simulink model "ME655_Grp7_Simulink_Latest"  (R2022b)
settings: Solver=FixedStepAuto  StartTime=0.0  StopTime=60  FixedStep=.003  RelTol=1e-3
values from neighbouring files (symbols this model uses):
  A = [1 T;0 1]    [ME655_Grp7_MATLAB.m]
  Bh = 62.8318530718    [ME655_Lect09_VL3_Data.mat]
  dt_active_control = 10    [ME655_Grp7_MATLAB.m]
  g = 9.81    [ME655_Lect09_VL3_Data.mat]
  h = 2.5*N    (= 200)    [ME655_Grp7_MATLAB.m]
  H = eye(2)    [ME655_Grp7_MATLAB.m]
  IHC = 1.16793611779    [ME655_Lect09_VL3_Data.mat]
  IRC = 0.090069676016    [ME655_Lect09_VL3_Data.mat]
  k = -K*RhipAvg + LhipAvg    [ME655_Grp7_MATLAB.m]
  K = Sp*C*inv(Sh)    [ME655_Grp7_MATLAB.m]
  Kh = 986.960440109    [ME655_Lect09_VL3_Data.mat]
  lambda = .95    (= 0.95)    [ME655_Grp7_MATLAB.m]
  LH = 0.426438    [ME655_Lect09_VL3_Data.mat]
  Lhip_pos0 = Lhip_pos(1)    [ME655_Grp7_MATLAB.m]
  Lhip_vel0 = Lhip_vel(1)    [ME655_Grp7_MATLAB.m]
  LR = 0.2474    [ME655_Lect09_VL3_Data.mat]
  M = 6    [ME655_Grp7_MATLAB.m]
  mH = 12.075    [ME655_Lect09_VL3_Data.mat]
  mR = 7.7284    [ME655_Lect09_VL3_Data.mat]
  N = 80    [ME655_Grp7_MATLAB.m]
  nu = .5    (= 0.5)    [ME655_Grp7_MATLAB.m]
  Q = G*G'*var(Lhip_acc(train_indices(:)))    [ME655_Grp7_MATLAB.m]
  R = [var(Lhip_pred(:,1)-Lhip_pos_train) 0;0 var(Lhip_pred(:,2)-Lhip_vel_train)]    [ME655_Grp7_MATLAB.m]
  t_start = 5.0    (= 5)    [ME655_Grp7_MATLAB.m]
  Tau_h_max = 30    [ME655_Grp7_MATLAB.m]
undefined symbols (not defined in the file or in its folder): theta_0, theta_d0
settings Model: Creator=Damiano  LastModifiedBy=peeratienthong
settings SolverCC: AlgebraicLoopSolver=TrustRegion
settings DataIOCC: ReturnWorkspaceOutputs=off
settings DebuggingCC: UnconnectedInputMsg=warning  UnconnectedOutputMsg=warning  UnconnectedLineMsg=warning  SFMachineParentedDataDiag=warning  ArithmeticOperatorsInVariantConditions=warning
settings ModelReferenceCC: EnableRefExpFcnMdlSchedulingChecks=on
settings SFSimCC: SimUseLocalCustomCode=off  CustomCodeUndefinedFunction=UseInterfaceOnly
settings RTWCC: RTWUseLocalCustomCode=off  DLArmComputeVersion=19.05
settings CodeAppCC: StateflowObjectComments=on

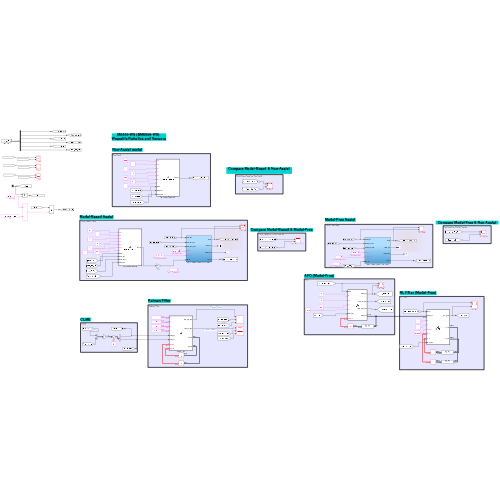
[thumbnail: Simulink's stored preview of the top-level diagram]
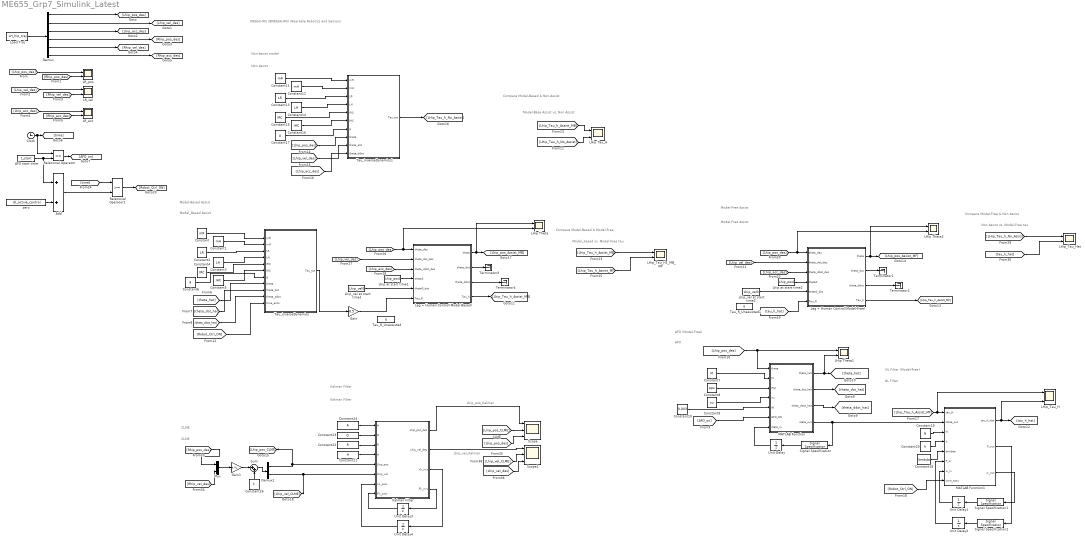
== system ME655_Grp7_Simulink_Latest ==
  note: Model_based vs. Model-Free tau
  note: Model-Free Assist
  note: NL Filter
  note: AFO
  note: Model_Based Assist
  note: Kalman Filter
  note: CLME
  note: Non Assist
  note: Model-Base Assist vs. Non Assist
  note: Lhip_pos_Kalman
  note: Lhip_vel_Kalman
  note: ME655-WS (BME656-WS)
      | Wearable Robotics and Sensors
  note: Non-Assist model
  note: Model-Based Assist
  note: Compare Model-Based & Non-Assist
  note: Model-Free Assist
  note: AFO (Model-Free)
  note: NL Filter (Model-Free)
  note: Compare Model-Based & Model-Free
  note: CLME
  note: Kalman Filter
  note: Compare Model-Free & Non Assist
  note: Non Assist vs. Model-Free tau
  AFO start time : Constant  Value=t_start
  Add : Sum
  Clock : Clock
  Constant : Constant  Value=mR
  Constant1 : Constant  Value=mH
  Constant10 : Constant  Value=0.003
  Constant11 : Constant  Value=mR
  Constant12 : Constant  Value=mH
  Constant13 : Constant  Value=LR
  Constant14 : Constant  Value=LH
  Constant15 : Constant  Value=IRC
  Constant16 : Constant  Value=IHC
  Constant17 : Constant  Value=g
  Constant18 : Constant  Value=lambda
  Constant19 : Constant  Value=N
  Constant2 : Constant  Value=LR
  Constant20 : Constant  Value=h
  Constant21 : Constant  Value=H
  Constant22 : Constant  Value=R
  Constant23 : Constant  Value=Q
  Constant24 : Constant  Value=A
  Constant26 : Constant  Value=k
  Constant3 : Constant  Value=LH
  Constant4 : Constant  Value=IRC
  Constant5 : Constant  Value=IHC
  Constant6 : Constant  Value=g
  Constant7 : Constant  Value=M
  Constant8 : Constant  Value=eps
  Constant9 : Constant  Value=nu
  Demux : Demux  Outputs=6
  Demux1 : Demux  Outputs=2
  Gain : Gain  Gain=0.5
  Gain1 : Gain  Gain=K  Multiplication=Matrix(K*u)
  Kalman Filter : MATLAB Function  TreatAsAtomicUnit=on
  LHip Tau_H : Scope  NumInputPorts=2
  LHip Theta : Scope  NumInputPorts=2
  LHip Theta1 : Scope  NumInputPorts=2
  LHip Theta2 : Scope  NumInputPorts=2
  LHip_Tau_H : Scope  NumInputPorts=2
  LHip_Tau_H1_MB_MF : Scope  NumInputPorts=2
  LHip_Tau_Hat : Scope  NumInputPorts=2
  "LR_acc " : Scope  NumInputPorts=2
  LR_pos : Scope  NumInputPorts=2
  LR_vel : Scope  NumInputPorts=2
  Leg + Human Control(Model-Based) : Subsystem
  Leg + Human Control(Model-Free) : Subsystem
  Lhip at start time1 : Constant  Value=Lhip_pos0
  Lhip at start time2 : Constant  Value=Lhip_pos0
  Lhip_vel at start time1 : Constant  Value=Lhip_vel0
  Lhip_vel at start time2 : Constant  Value=Lhip_vel0
  Load Traj : FromWorkspace  VariableName=LH_hip_traj
  MATLAB Function : MATLAB Function  TreatAsAtomicUnit=on
  MATLAB Function1 : MATLAB Function  TreatAsAtomicUnit=on
  Mux : Mux  Inputs=2
  Relational Operator : RelationalOperator  OutDataTypeStr=boolean  RndMeth=Simplest  InputSameDT=off
  Relational Operator1 : RelationalOperator  OutDataTypeStr=boolean  RndMeth=Simplest  InputSameDT=off
  Scope : Scope  NumInputPorts=3
  Scope1 : Scope  NumInputPorts=3
  Signal Specification : SignalSpecification  Dimensions=[1,14]
  Signal Specification1 : SignalSpecification  Dimensions=[1,N]
  Signal Specification2 : SignalSpecification  Dimensions=[1,N]
  Sum : Sum  Inputs=|++
  Tau_R_Unassisted : Constant  Value=0
  Tau_R_Unassisted1 : Constant  Value=0
  Tau_inverseDynamics : MATLAB Function  TreatAsAtomicUnit=on
  Tau_inverseDynamics1 : MATLAB Function  TreatAsAtomicUnit=on
  Terminator{1..4} (4 alike) : Terminator
  Unit Delay : UnitDelay  InitialCondition=[[pi/2,pi/2,pi/2,pi/2,pi/2,pi/2],[0,0,0,0,0,0], 3*pi/2, 0]  SampleTime=-1  HasFrameUpgradeWarning=on
  Unit Delay1 : UnitDelay  InitialCondition=zeros(1,N)  SampleTime=-1  HasFrameUpgradeWarning=on
  Unit Delay2 : UnitDelay  InitialCondition=ones(1,N)  SampleTime=-1  HasFrameUpgradeWarning=on
  Unit Delay3 : UnitDelay  InitialCondition=eye(2)  SampleTime=-1  HasFrameUpgradeWarning=on
  Unit Delay4 : UnitDelay  InitialCondition=[0;0]  SampleTime=-1  HasFrameUpgradeWarning=on
  zero : Constant  Value=dt_active_control
  wires:
  Load Traj/1 -> Demux/1
  Demux/6 -> [Rhip_acc_des]
  Demux/4 -> [Rhip_pos_des]
  Demux/5 -> [Rhip_vel_des]
  [Lhip_pos_des] -> LR_pos/1
  [Rhip_pos_des] -> LR_pos/2
  [Lhip_vel_des] -> LR_vel/1
  [Rhip_vel_des] -> LR_vel/2
  [Lhip_acc_des] -> "LR_acc "/1
  [Rhip_acc_des] -> "LR_acc "/2
  Clock/1 -> Relational Operator/1, [time]
  Relational Operator/1 -> [AFO_on]
  [time] -> Relational Operator1/1
  AFO start time/1 -> Add/1, Relational Operator/2
  Add/1 -> Relational Operator1/2
  zero/1 -> Add/2
  [Lhip_acc_des] -> Leg + Human Control(Model-Based)/3(theta_ddot_des)
  Leg + Human Control(Model-Based)/3(theta_ddot) -> Terminator4/1
  Lhip_vel at start time1/1 -> Leg + Human Control(Model-Based)/5(theta0_dot)
  Leg + Human Control(Model-Based)/2(theta_dot) -> Terminator3/1
  [Lhip_vel_des] -> Leg + Human Control(Model-Based)/2(theta_dot_des)
  Lhip at start time1/1 -> Leg + Human Control(Model-Based)/4(theta0)
  Leg + Human Control(Model-Based)/4(Tau_h) -> [Lhip_Tau_h_Assist_MB]
  [Lhip_pos_des] -> Leg + Human Control(Model-Based)/1(theta_des), LHip Theta/2
  Relational Operator1/1 -> [Robot_Ctrl_ON]
  Demux/1 -> [Lhip_pos_des]
  Demux/2 -> [Lhip_vel_des]
  Demux/3 -> [Lhip_acc_des]
  [theta_hat] -> Tau_inverseDynamics/8(theta)
  [theta_dot_hat] -> Tau_inverseDynamics/9(theta_dot)
  [theta_ddot_hat] -> Tau_inverseDynamics/10(theta_ddot)
  Constant/1 -> Tau_inverseDynamics/1(mR)
  Constant1/1 -> Tau_inverseDynamics/2(mH)
  Constant2/1 -> Tau_inverseDynamics/3(LR)
  Constant3/1 -> Tau_inverseDynamics/4(LH)
  Constant4/1 -> Tau_inverseDynamics/5(IRC)
  Constant5/1 -> Tau_inverseDynamics/6(IHC)
  Constant6/1 -> Tau_inverseDynamics/7(g)
  [AFO_on] -> MATLAB Function/6(AFO_ON)
  Constant9/1 -> MATLAB Function/4(nu)
  Constant8/1 -> MATLAB Function/3(esp)
  Constant7/1 -> MATLAB Function/2(M)
  [Lhip_pos_des] -> LHip Theta1/1, MATLAB Function/1(theta)
  MATLAB Function/1(theta_hat) -> [theta_hat], LHip Theta1/2
  Leg + Human Control(Model-Based)/1(theta) -> LHip Theta/1, [Lhip_pos_Assist_MB]
  Constant10/1 -> MATLAB Function/5(dt)
  MATLAB Function/3(theta_ddot_hat) -> [theta_ddot_hat]
  MATLAB Function/2(theta_dot_hat) -> [theta_dot_hat]
  Unit Delay/1 -> MATLAB Function/7(state_in)
  Signal Specification/1 -> Unit Delay/1
  MATLAB Function/4(state_out) -> MATLAB Function1/2(state_out), Signal Specification/1
  [Robot_Ctrl_ON] -> Tau_inverseDynamics/11(time_activ)
  [Lhip_pos_des] -> Tau_inverseDynamics1/8(theta)
  Constant13/1 -> Tau_inverseDynamics1/3(LR)
  Constant11/1 -> Tau_inverseDynamics1/1(mR)
  Constant12/1 -> Tau_inverseDynamics1/2(mH)
  Constant14/1 -> Tau_inverseDynamics1/4(LH)
  Constant15/1 -> Tau_inverseDynamics1/5(IRC)
  [Lhip_acc_des] -> Tau_inverseDynamics1/10(theta_ddot)
  Constant17/1 -> Tau_inverseDynamics1/7(g)
  [Lhip_vel_des] -> Tau_inverseDynamics1/9(theta_dot)
  Constant16/1 -> Tau_inverseDynamics1/6(IHC)
  Tau_inverseDynamics1/1(Tau_tot) -> [LHip_Tau_h_No_Assist]
  Tau_inverseDynamics/1(Tau_tot) -> Gain/1
  [Lhip_Tau_h_Assist_MB] -> LHip Tau_H/1
  [LHip_Tau_h_No_Assist] -> LHip Tau_H/2
  Signal Specification1/1 -> Unit Delay1/1
  Signal Specification2/1 -> Unit Delay2/1
  MATLAB Function1/3(w_out) -> Signal Specification1/1
  MATLAB Function1/2(P_out) -> Signal Specification2/1
  Unit Delay1/1 -> MATLAB Function1/7(w_in)
  Unit Delay2/1 -> MATLAB Function1/6(P_in)
  Constant19/1 -> MATLAB Function1/3(N)
  Constant20/1 -> MATLAB Function1/4(h)
  Constant18/1 -> MATLAB Function1/5(lambda)
  [Lhip_Tau_h_Assist_MF] -> LHip_Tau_H/1, MATLAB Function1/1(tau_H)
  MATLAB Function1/1(tau_h_hat) -> LHip_Tau_H/2, [tau_h_hat]
  [Robot_Ctrl_ON] -> MATLAB Function1/8(time_activ)
  Leg + Human Control(Model-Free)/4(Tau_h) -> [Lhip_Tau_h_Assist_MF]
  Leg + Human Control(Model-Free)/2(theta_dot) -> Terminator1/1
  Leg + Human Control(Model-Free)/3(theta_ddot) -> Terminator2/1
  [Lhip_vel_des] -> Leg + Human Control(Model-Free)/2(theta_dot_des)
  Lhip at start time2/1 -> Leg + Human Control(Model-Free)/4(theta0)
  Leg + Human Control(Model-Free)/1(theta) -> LHip Theta2/1, [Lhip_pos_Assist_MF]
  [Lhip_acc_des] -> Leg + Human Control(Model-Free)/3(theta_ddot_des)
  Lhip_vel at start time2/1 -> Leg + Human Control(Model-Free)/5(theta0_dot)
  [Lhip_pos_des] -> Leg + Human Control(Model-Free)/1(theta_des), LHip Theta2/2
  [Lhip_Tau_h_Assist_MF] -> LHip_Tau_H1_MB_MF/2
  [Lhip_Tau_h_Assist_MB] -> LHip_Tau_H1_MB_MF/1
  Constant24/1 -> Kalman Filter/1(A)
  Constant23/1 -> Kalman Filter/2(Q)
  Constant22/1 -> Kalman Filter/3(R)
  Constant21/1 -> Kalman Filter/4(H)
  [Rhip_pos_des] -> Mux/1
  [Rhip_vel_des] -> Mux/2
  Mux/1 -> Gain1/1
  Gain1/1 -> Sum/1
  Constant26/1 -> Sum/2
  Sum/1 -> Demux1/1
  Demux1/1 -> Kalman Filter/5(Lhip_pos), [Lhip_pos_CLME]
  Demux1/2 -> [Lhip_vel_CLME], Kalman Filter/6(Lhip_vel)
  Unit Delay3/1 -> Kalman Filter/8(Pk_prev)
  Kalman Filter/4(Pk_nxt) -> Unit Delay3/1
  Kalman Filter/3(xk_nxt) -> Unit Delay4/1
  Unit Delay4/1 -> Kalman Filter/7(xk_prev)
  Kalman Filter/1(Lhip_pos_des) -> Scope/1
  Kalman Filter/2(Lhip_vel_des) -> Scope1/1
  [Lhip_pos_des] -> Scope/3
  [Lhip_vel_des] -> Scope1/3
  [Lhip_pos_CLME] -> Scope/2
  [Lhip_vel_CLME] -> Scope1/2
  Gain/1 -> Leg + Human Control(Model-Based)/6(Tau_R)
  [LHip_Tau_h_No_Assist] -> LHip_Tau_Hat/1
  [tau_h_hat] -> LHip_Tau_Hat/2
  [tau_h_hat] -> Leg + Human Control(Model-Free)/6(Tau_R)

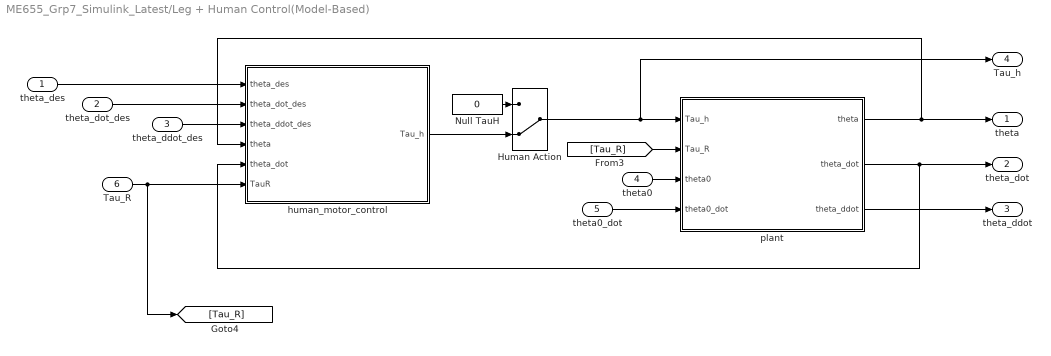
== system ME655_Grp7_Simulink_Latest/Leg + Human Control(Model-Based) ==
  theta_des : Inport
  theta_dot_des : Inport  Port=2
  theta_ddot_des : Inport  Port=3
  theta0 : Inport  Port=4
  theta0_dot : Inport  Port=5
  Tau_R : Inport  Port=6
  Human Action : ManualSwitch  CurrentSetting=0
  Null TauH : Constant  Value=0
  human_motor_control : Subsystem
  plant : Subsystem
  theta : Outport  PortDimensions=[1,1]  VectorParamsAs1DForOutWhenUnconnected=off
  theta_dot : Outport  Port=2  PortDimensions=[1,1]  VectorParamsAs1DForOutWhenUnconnected=off
  theta_ddot : Outport  Port=3  PortDimensions=[1,1]  VectorParamsAs1DForOutWhenUnconnected=off
  Tau_h : Outport  Port=4  PortDimensions=[1,1]  VectorParamsAs1DForOutWhenUnconnected=off
  wires:
  theta_des/1 -> human_motor_control/1(theta_des)
  theta_dot_des/1 -> human_motor_control/2(theta_dot_des)
  theta0/1 -> plant/3(theta0)
  theta0_dot/1 -> plant/4(theta0_dot)
  [Tau_R] -> plant/2(Tau_R)
  plant/1(theta) -> theta/1, human_motor_control/4(theta)
  plant/2(theta_dot) -> human_motor_control/5(theta_dot), theta_dot/1
  plant/3(theta_ddot) -> theta_ddot/1
  theta_ddot_des/1 -> human_motor_control/3(theta_ddot_des)
  human_motor_control/1(Tau_h) -> Human Action/2
  Human Action/1 -> Tau_h/1, plant/1(Tau_h)
  Null TauH/1 -> Human Action/1
  Tau_R/1 -> [Tau_R], human_motor_control/6(TauR)

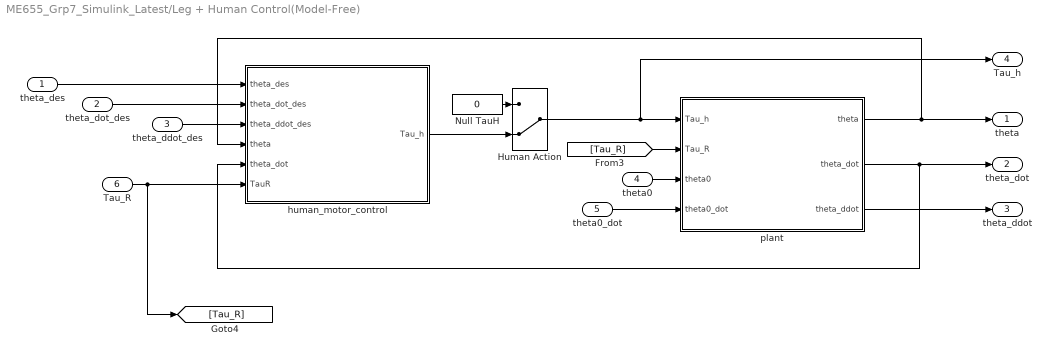
== system ME655_Grp7_Simulink_Latest/Leg + Human Control(Model-Free) ==
  theta_des : Inport
  theta_dot_des : Inport  Port=2
  theta_ddot_des : Inport  Port=3
  theta0 : Inport  Port=4
  theta0_dot : Inport  Port=5
  Tau_R : Inport  Port=6
  Human Action : ManualSwitch  CurrentSetting=0
  Null TauH : Constant  Value=0
  human_motor_control : Subsystem
  plant : Subsystem
  theta : Outport  PortDimensions=[1,1]  VectorParamsAs1DForOutWhenUnconnected=off
  theta_dot : Outport  Port=2  PortDimensions=[1,1]  VectorParamsAs1DForOutWhenUnconnected=off
  theta_ddot : Outport  Port=3  PortDimensions=[1,1]  VectorParamsAs1DForOutWhenUnconnected=off
  Tau_h : Outport  Port=4  PortDimensions=[1,1]  VectorParamsAs1DForOutWhenUnconnected=off
  wires:
  theta_des/1 -> human_motor_control/1(theta_des)
  theta_dot_des/1 -> human_motor_control/2(theta_dot_des)
  theta0/1 -> plant/3(theta0)
  theta0_dot/1 -> plant/4(theta0_dot)
  [Tau_R] -> plant/2(Tau_R)
  plant/1(theta) -> theta/1, human_motor_control/4(theta)
  plant/2(theta_dot) -> human_motor_control/5(theta_dot), theta_dot/1
  plant/3(theta_ddot) -> theta_ddot/1
  theta_ddot_des/1 -> human_motor_control/3(theta_ddot_des)
  human_motor_control/1(Tau_h) -> Human Action/2
  Human Action/1 -> Tau_h/1, plant/1(Tau_h)
  Null TauH/1 -> Human Action/1
  Tau_R/1 -> [Tau_R], human_motor_control/6(TauR)

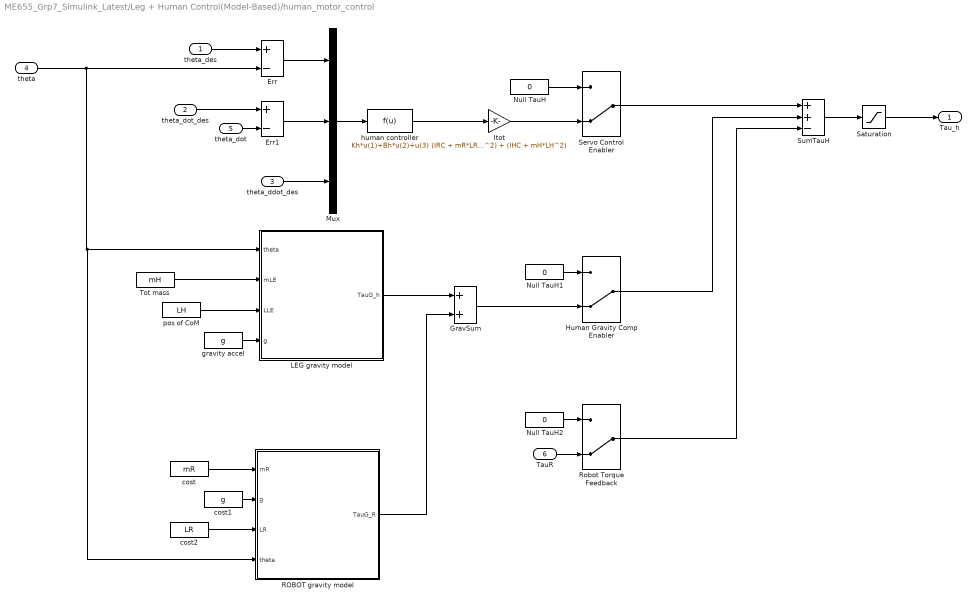
== system ME655_Grp7_Simulink_Latest/Leg + Human Control(Model-Based)/human_motor_control ==
  theta_des : Inport
  theta_dot_des : Inport  Port=2
  theta_ddot_des : Inport  Port=3
  theta : Inport  Port=4
  theta_dot : Inport  Port=5
  TauR : Inport  Port=6
  Err : Sum  Inputs=+-
  Err1 : Sum  Inputs=+-
  GravSum : Sum
  Human Gravity Comp Enabler : ManualSwitch  CurrentSetting=0
  Itot : Gain  Gain=(IRC + mR*LR^2) + (IHC + mH*LH^2)
  LEG gravity model : MATLAB Function  TreatAsAtomicUnit=on
  Mux : Mux  Inputs=3
  Null TauH : Constant  Value=0
  Null TauH1 : Constant  Value=0
  Null TauH2 : Constant  Value=0
  ROBOT gravity model : MATLAB Function  TreatAsAtomicUnit=on
  Robot Torque Feedback : ManualSwitch  CurrentSetting=0
  Saturation : Saturate  UpperLimit=Tau_h_max  LowerLimit=-Tau_h_max
  Servo Control Enabler : ManualSwitch  CurrentSetting=0
  SumTauH : Sum  Inputs=++-
  Tot mass : Constant  Value=mH
  cost : Constant  Value=mR
  cost1 : Constant  Value=g
  cost2 : Constant  Value=LR
  gravity accel : Constant  Value=g
  human controller : Fcn  Expr=Kh*u(1)+Bh*u(2)+u(3)
  pos of CoM : Constant  Value=LH
  Tau_h : Outport  PortDimensions=[1,1]  VectorParamsAs1DForOutWhenUnconnected=off
  wires:
  theta_des/1 -> Err/1
  theta_dot_des/1 -> Err1/1
  theta_dot/1 -> Err1/2
  Err/1 -> Mux/1
  Err1/1 -> Mux/2
  Mux/1 -> human controller/1
  theta_ddot_des/1 -> Mux/3
  gravity accel/1 -> LEG gravity model/4(g)
  Tot mass/1 -> LEG gravity model/2(mLE)
  pos of CoM/1 -> LEG gravity model/3(LLE)
  Null TauH/1 -> Servo Control Enabler/1
  Null TauH1/1 -> Human Gravity Comp Enabler/1
  Human Gravity Comp Enabler/1 -> SumTauH/2
  SumTauH/1 -> Saturation/1
  human controller/1 -> Itot/1
  Servo Control Enabler/1 -> SumTauH/1
  Saturation/1 -> Tau_h/1
  Itot/1 -> Servo Control Enabler/2
  Null TauH2/1 -> Robot Torque Feedback/1
  TauR/1 -> Robot Torque Feedback/2
  Robot Torque Feedback/1 -> SumTauH/3
  theta/1 -> ROBOT gravity model/4(theta), LEG gravity model/1(theta), Err/2
  ROBOT gravity model/1(TauG_R) -> GravSum/2
  cost2/1 -> ROBOT gravity model/3(LR)
  cost/1 -> ROBOT gravity model/1(mR)
  cost1/1 -> ROBOT gravity model/2(g)
  LEG gravity model/1(TauG_h) -> GravSum/1
  GravSum/1 -> Human Gravity Comp Enabler/2

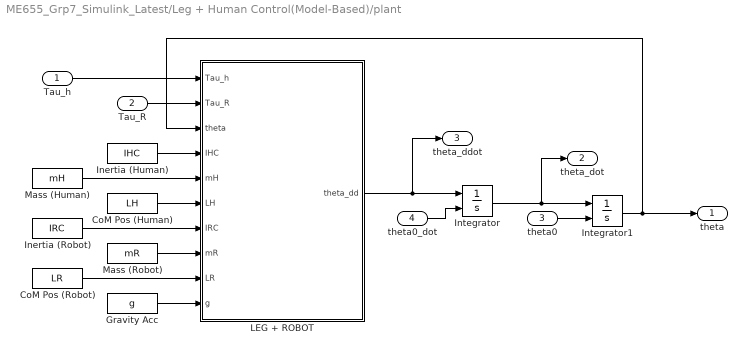
== system ME655_Grp7_Simulink_Latest/Leg + Human Control(Model-Based)/plant ==
  Tau_h : Inport
  Tau_R : Inport  Port=2
  theta0 : Inport  Port=3
  theta0_dot : Inport  Port=4
  CoM Pos (Human) : Constant  Value=LH
  CoM Pos (Robot) : Constant  Value=LR
  Gravity Acc : Constant  Value=g
  Inertia (Human) : Constant  Value=IHC
  Inertia (Robot) : Constant  Value=IRC
  Integrator : Integrator  InitialConditionSource=external  InitialCondition=theta_d0
  Integrator1 : Integrator  InitialConditionSource=external  InitialCondition=theta_0
  LEG + ROBOT : MATLAB Function  TreatAsAtomicUnit=on
  Mass (Human) : Constant  Value=mH
  Mass (Robot) : Constant  Value=mR
  theta : Outport  PortDimensions=[1,1]  VectorParamsAs1DForOutWhenUnconnected=off
  theta_dot : Outport  Port=2  PortDimensions=[1,1]  VectorParamsAs1DForOutWhenUnconnected=off
  theta_ddot : Outport  Port=3  PortDimensions=[1,1]  VectorParamsAs1DForOutWhenUnconnected=off
  wires:
  Tau_h/1 -> LEG + ROBOT/1(Tau_h)
  Tau_R/1 -> LEG + ROBOT/2(Tau_R)
  LEG + ROBOT/1(theta_dd) -> theta_ddot/1, Integrator/1
  Integrator/1 -> theta_dot/1, Integrator1/1
  theta0_dot/1 -> Integrator/2
  theta0/1 -> Integrator1/2
  Integrator1/1 -> LEG + ROBOT/3(theta), theta/1
  Inertia (Human)/1 -> LEG + ROBOT/4(IHC)
  Mass (Human)/1 -> LEG + ROBOT/5(mH)
  CoM Pos (Human)/1 -> LEG + ROBOT/6(LH)
  Gravity Acc/1 -> LEG + ROBOT/10(g)
  Mass (Robot)/1 -> LEG + ROBOT/8(mR)
  CoM Pos (Robot)/1 -> LEG + ROBOT/9(LR)
  Inertia (Robot)/1 -> LEG + ROBOT/7(IRC)

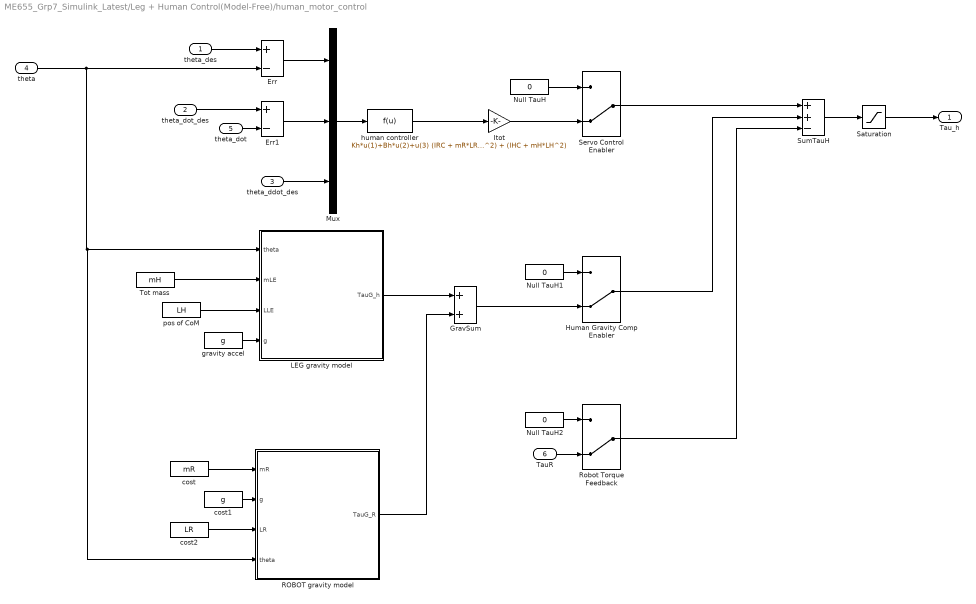
== system ME655_Grp7_Simulink_Latest/Leg + Human Control(Model-Free)/human_motor_control ==
  theta_des : Inport
  theta_dot_des : Inport  Port=2
  theta_ddot_des : Inport  Port=3
  theta : Inport  Port=4
  theta_dot : Inport  Port=5
  TauR : Inport  Port=6
  Err : Sum  Inputs=+-
  Err1 : Sum  Inputs=+-
  GravSum : Sum
  Human Gravity Comp Enabler : ManualSwitch  CurrentSetting=0
  Itot : Gain  Gain=(IRC + mR*LR^2) + (IHC + mH*LH^2)
  LEG gravity model : MATLAB Function  TreatAsAtomicUnit=on
  Mux : Mux  Inputs=3
  Null TauH : Constant  Value=0
  Null TauH1 : Constant  Value=0
  Null TauH2 : Constant  Value=0
  ROBOT gravity model : MATLAB Function  TreatAsAtomicUnit=on
  Robot Torque Feedback : ManualSwitch  CurrentSetting=0
  Saturation : Saturate  UpperLimit=Tau_h_max  LowerLimit=-Tau_h_max
  Servo Control Enabler : ManualSwitch  CurrentSetting=0
  SumTauH : Sum  Inputs=++-
  Tot mass : Constant  Value=mH
  cost : Constant  Value=mR
  cost1 : Constant  Value=g
  cost2 : Constant  Value=LR
  gravity accel : Constant  Value=g
  human controller : Fcn  Expr=Kh*u(1)+Bh*u(2)+u(3)
  pos of CoM : Constant  Value=LH
  Tau_h : Outport  PortDimensions=[1,1]  VectorParamsAs1DForOutWhenUnconnected=off
  wires:
  theta_des/1 -> Err/1
  theta_dot_des/1 -> Err1/1
  theta_dot/1 -> Err1/2
  Err/1 -> Mux/1
  Err1/1 -> Mux/2
  Mux/1 -> human controller/1
  theta_ddot_des/1 -> Mux/3
  gravity accel/1 -> LEG gravity model/4(g)
  Tot mass/1 -> LEG gravity model/2(mLE)
  pos of CoM/1 -> LEG gravity model/3(LLE)
  Null TauH/1 -> Servo Control Enabler/1
  Null TauH1/1 -> Human Gravity Comp Enabler/1
  Human Gravity Comp Enabler/1 -> SumTauH/2
  SumTauH/1 -> Saturation/1
  human controller/1 -> Itot/1
  Servo Control Enabler/1 -> SumTauH/1
  Saturation/1 -> Tau_h/1
  Itot/1 -> Servo Control Enabler/2
  Null TauH2/1 -> Robot Torque Feedback/1
  TauR/1 -> Robot Torque Feedback/2
  Robot Torque Feedback/1 -> SumTauH/3
  theta/1 -> ROBOT gravity model/4(theta), LEG gravity model/1(theta), Err/2
  ROBOT gravity model/1(TauG_R) -> GravSum/2
  cost2/1 -> ROBOT gravity model/3(LR)
  cost/1 -> ROBOT gravity model/1(mR)
  cost1/1 -> ROBOT gravity model/2(g)
  LEG gravity model/1(TauG_h) -> GravSum/1
  GravSum/1 -> Human Gravity Comp Enabler/2

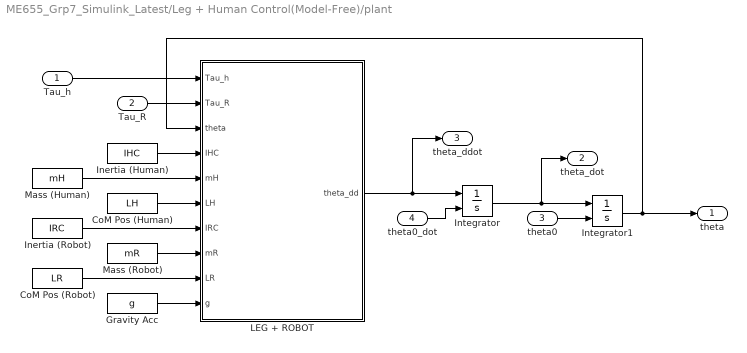
== system ME655_Grp7_Simulink_Latest/Leg + Human Control(Model-Free)/plant ==
  Tau_h : Inport
  Tau_R : Inport  Port=2
  theta0 : Inport  Port=3
  theta0_dot : Inport  Port=4
  CoM Pos (Human) : Constant  Value=LH
  CoM Pos (Robot) : Constant  Value=LR
  Gravity Acc : Constant  Value=g
  Inertia (Human) : Constant  Value=IHC
  Inertia (Robot) : Constant  Value=IRC
  Integrator : Integrator  InitialConditionSource=external  InitialCondition=theta_d0
  Integrator1 : Integrator  InitialConditionSource=external  InitialCondition=theta_0
  LEG + ROBOT : MATLAB Function  TreatAsAtomicUnit=on
  Mass (Human) : Constant  Value=mH
  Mass (Robot) : Constant  Value=mR
  theta : Outport  PortDimensions=[1,1]  VectorParamsAs1DForOutWhenUnconnected=off
  theta_dot : Outport  Port=2  PortDimensions=[1,1]  VectorParamsAs1DForOutWhenUnconnected=off
  theta_ddot : Outport  Port=3  PortDimensions=[1,1]  VectorParamsAs1DForOutWhenUnconnected=off
  wires:
  Tau_h/1 -> LEG + ROBOT/1(Tau_h)
  Tau_R/1 -> LEG + ROBOT/2(Tau_R)
  LEG + ROBOT/1(theta_dd) -> theta_ddot/1, Integrator/1
  Integrator/1 -> theta_dot/1, Integrator1/1
  theta0_dot/1 -> Integrator/2
  theta0/1 -> Integrator1/2
  Integrator1/1 -> LEG + ROBOT/3(theta), theta/1
  Inertia (Human)/1 -> LEG + ROBOT/4(IHC)
  Mass (Human)/1 -> LEG + ROBOT/5(mH)
  CoM Pos (Human)/1 -> LEG + ROBOT/6(LH)
  Gravity Acc/1 -> LEG + ROBOT/10(g)
  Mass (Robot)/1 -> LEG + ROBOT/8(mR)
  CoM Pos (Robot)/1 -> LEG + ROBOT/9(LR)
  Inertia (Robot)/1 -> LEG + ROBOT/7(IRC)

== matlab function ME655_Grp7_Simulink_Latest/Leg + Human Control(Model-Free)/plant/LEG + ROBOT ==
  data: Tau_h input; Tau_R input; theta input; theta_dd output; IHC input; mH input; LH input; IRC input; mR input; LR input; g input
function theta_dd   = LegRobotModel(Tau_h,Tau_R,theta,IHC,mH,LH,IRC,mR,LR,g)

theta_dd = 1/((IRC + mR*LR^2)+(IHC + mH*LH^2)) * (Tau_h-mH*g*LH*sin(theta) + Tau_R-mR*g*LR*sin(theta));

end

== matlab function ME655_Grp7_Simulink_Latest/Leg + Human Control(Model-Based)/human_motor_control/LEG gravity model ==
  data: theta input; mLE input; LLE input; TauG_h output; g input
function TauG_h   = HumanLegGravModel(theta,mLE,LLE,g)
% human gravity compensation term
TauG_h=mLE*g*LLE*sin(theta);

end

== matlab function ME655_Grp7_Simulink_Latest/Kalman Filter ==
  data: A input; Lhip_pos_des output; Q input; R input; H input; Lhip_pos input; Lhip_vel input; xk_prev input; Pk_prev input; Lhip_vel_des output; xk_nxt output; Pk_nxt output
function [Lhip_pos_des, Lhip_vel_des, xk_nxt, Pk_nxt] = KF(A,Q,R,H,Lhip_pos,Lhip_vel,xk_prev,Pk_prev)
    
    zk = [Lhip_pos;Lhip_vel];
    %prediction stage
    xk_pred = A*xk_prev;
    Pk_pred = A*Pk_prev*A' + Q;
    
    %correction stage
    K = Pk_pred*H'*inv(H*Pk_pred*H' + R);
    xk_nxt = xk_pred + K*(zk - H*xk_prev);
    Pk_nxt = (eye(2) - K*H)*Pk_pred;

    Lhip_pos_des = xk_nxt(1);
    Lhip_vel_des = xk_nxt(2);
end

== matlab function ME655_Grp7_Simulink_Latest/Leg + Human Control(Model-Based)/human_motor_control/ROBOT gravity model ==
  data: mR input; g input; LR input; theta input; TauG_R output
function TauG_R  = RobotGravModel(mR,g,LR,theta)

TauG_R=mR*g*LR*sin(theta);
% TauG_h=mLE*g*LLE*sin(theta);

end

== matlab function ME655_Grp7_Simulink_Latest/Leg + Human Control(Model-Based)/plant/LEG + ROBOT ==
  data: Tau_h input; Tau_R input; theta input; theta_dd output; IHC input; mH input; LH input; IRC input; mR input; LR input; g input
function theta_dd   = LegRobotModel(Tau_h,Tau_R,theta,IHC,mH,LH,IRC,mR,LR,g)

theta_dd = 1/((IRC + mR*LR^2)+(IHC + mH*LH^2)) * (Tau_h-mH*g*LH*sin(theta) + Tau_R-mR*g*LR*sin(theta));

end

== matlab function ME655_Grp7_Simulink_Latest/MATLAB Function ==
  data: theta input; theta_hat output; M input; esp input; nu input; dt input; AFO_ON input; state_in input; theta_dot_hat output; theta_ddot_hat output; state_out output
function [theta_hat, theta_dot_hat, theta_ddot_hat, state_out] = AFO(theta, M, esp, nu, dt, AFO_ON, state_in)
%Mvec = 1:1:M; %create a vector of harmonic signals
%state_in [Phi; a; w; theta0]
Phi = state_in(1:6);
a = state_in(7:12);
w = state_in(13);
theta0 = state_in(14);

if AFO_ON
    
    sumF = 0;
    for m=1:M
        sumF = sumF + a(m)*sin(Phi(m));
    end
    %error signal
    F = theta - theta0 - sumF;
    %update state
    for j=1:M
        Phi(j) = mod(Phi(j)+dt*(j*w+esp*F*cos(Phi(j))),2*pi);
        a(j) = a(j)+dt*nu*F*sin(Phi(j));
    end
    w = w+dt*esp*F*cos(Phi(1));
    theta0 = theta0+dt*nu*F;
    %assign to state_out
    state_out = [Phi, a, w, theta0];

    %update est.
    sm1 = 0; sm2 = 0; sm3 = 0;
    for i=1:M
        sm1 = sm1 + a(i)*sin(Phi(i));
        sm2 = sm2 + i*w*a(i)*cos(Phi(i));
        sm3 = sm3 - i*power(w,2)*a(i)*sin(Phi(i)); 
    end
    theta_hat = theta0+sm1;
    theta_dot_hat = sm2;
    theta_ddot_hat = sm3;
   
else
    state_out = state_in;
 
    %update est.
    theta_hat = 0;
    theta_dot_hat = 0;
    theta_ddot_hat = 0;
end


end

== matlab function ME655_Grp7_Simulink_Latest/Tau_inverseDynamics ==
  data: mR input; Tau_tot output; mH input; LR input; LH input; IRC input; IHC input; g input; theta input; theta_dot input; theta_ddot input; time_activ input
function Tau_tot = inverse_dynamics(mR, mH, LR, LH, IRC, IHC, g, theta, theta_dot, theta_ddot, time_activ)
    
    if time_activ

        I_tot = (IRC+mR*LR^2) + (IHC+mH*LH^2);
        Tau_tot = I_tot*theta_ddot + mR*g*LR*sin(theta) + mH*g*LH*sin(theta);
    else
        Tau_tot = 0;
end

== matlab function ME655_Grp7_Simulink_Latest/Tau_inverseDynamics1 ==
  data: mR input; Tau_tot output; mH input; LR input; LH input; IRC input; IHC input; g input; theta input; theta_dot input; theta_ddot input
function Tau_tot = inverse_dynamics(mR, mH, LR, LH, IRC, IHC, g, theta, theta_dot, theta_ddot)

    I_tot = (IRC+mR*LR^2) + (IHC+mH*LH^2);
    Tau_tot = I_tot*theta_ddot + mR*g*LR*sin(theta) + mH*g*LH*sin(theta);
    
end

== matlab function ME655_Grp7_Simulink_Latest/MATLAB Function1 ==
  data: tau_H input; tau_h_hat output; state_out input; N input; h input; lambda input; P_in input; w_in input; P_out output; w_out output; time_activ input
function [tau_h_hat,P_out,w_out] = NL_filter(tau_H, state_out, N, h, lambda, P_in, w_in, time_activ)
    
    if time_activ
        %define variable & state
        phi_1 = state_out(1);
        kernel = zeros(size(P_in));
        kernel_weighted_sum = zeros(size(P_in));
        P_out = zeros(size(P_in));
        w_out = zeros(size(w_in));
        
        %define error signal
        e = zeros(size(w_in));
        for i = 1:N
            %error signal assignment
            e(i) = tau_H - w_in(i);
            kernel(i) = exp(h*(cos(phi_1-2*pi*i/N)-1));
            kernel_weighted_sum(i) = kernel(i)*w_in(i);
        end
        
        %estimate tau_h
        tau_h_hat = kernel_weighted_sum/kernel;
        
        for j = 1:N
            %update state
            P_out(j) = (1/lambda)*(P_in(j) - P_in(j)^2/(lambda/kernel(j)+P_in(j)));
            w_out(j) = w_in(j) + kernel(j)*P_out(j)*e(j);
        end

    else
        tau_h_hat = 0;
        P_out = P_in;
        w_out = w_in;
    end


end

== matlab function ME655_Grp7_Simulink_Latest/Leg + Human Control(Model-Free)/human_motor_control/LEG gravity model ==
  data: theta input; mLE input; LLE input; TauG_h output; g input
function TauG_h   = HumanLegGravModel(theta,mLE,LLE,g)
% human gravity compensation term
TauG_h=mLE*g*LLE*sin(theta);

end

== matlab function ME655_Grp7_Simulink_Latest/Leg + Human Control(Model-Free)/human_motor_control/ROBOT gravity model ==
  data: mR input; g input; LR input; theta input; TauG_R output
function TauG_R  = RobotGravModel(mR,g,LR,theta)

TauG_R=mR*g*LR*sin(theta);
% TauG_h=mLE*g*LLE*sin(theta);

end
